simulink subsystem "Gcm"  (R2021b)
settings: Solver=VariableStepAuto  StartTime=0.0  StopTime=10.0  RelTol=1e-3
undefined symbols (not defined in the file): Gcm_den_s1_SM_3, Gcm_den_s2_SM_3, K_SM_3
settings Model: Creator=sama1402  LastModifiedBy=sama1402

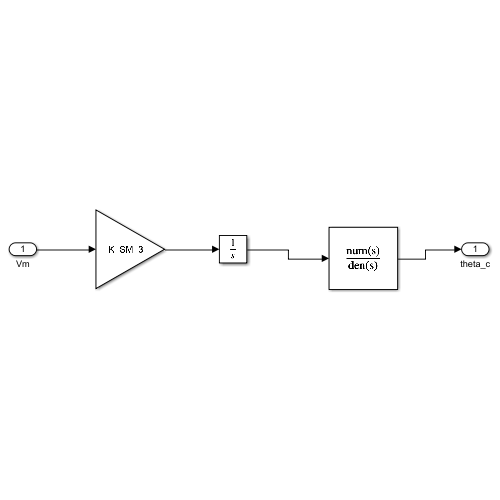
[thumbnail: Simulink's stored preview of the top-level diagram]
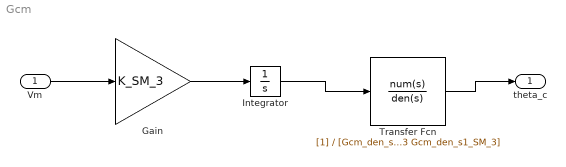
== system Gcm ==
  Vm : Inport
  Gain : Gain  Gain=K_SM_3
  Integrator : Integrator
  Transfer Fcn : TransferFcn  Denominator=[Gcm_den_s2_SM_3 Gcm_den_s1_SM_3]
  theta_c : Outport
  wires:
  Transfer Fcn/1 -> theta_c/1
  Integrator/1 -> Transfer Fcn/1
  Gain/1 -> Integrator/1
  Vm/1 -> Gain/1
